simulink model "S1"  (R2023b)
settings: Solver=FixedStepAuto  StartTime=0.0  StopTime=Time-Step_T  FixedStep=Step_T  RelTol=1e-3
InitFcn:
  | run("P_sim.m")
values from neighbouring files (symbols this model uses):
  Step_T = 0.001    [P_sim.m]
  T = 0.1    [P_sim.m]
  x_1_0 = 0.2    [P_sim.m]
  x_2_0 = 0.5    [P_sim.m]
  x_3_0 = -1    [P_sim.m]
undefined symbols (not defined in the file or in its folder): pam
settings Model: Creator=admin  LastModifiedBy=admin

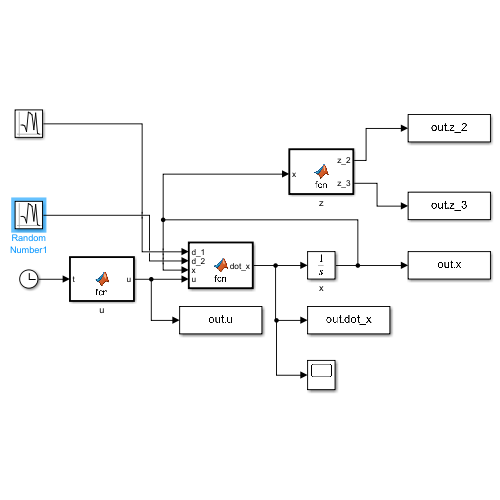
[thumbnail: Simulink's stored preview of the top-level diagram]
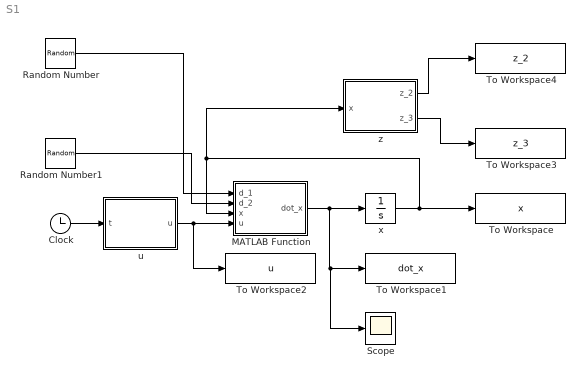
== system S1 ==
  Clock : Clock
  MATLAB Function : MATLAB Function  TreatAsAtomicUnit=on
  Random Number : RandomNumber  Variance=pam.d*pam.d  Seed=-1  SampleTime=Step_T
  Random Number1 : RandomNumber  Variance=pam.d*pam.d  Seed=1  SampleTime=Step_T
  Scope : Scope
  To Workspace : ToWorkspace  VariableName=x  SaveFormat=Timeseries  SampleTime=T
  To Workspace1 : ToWorkspace  VariableName=dot_x  SaveFormat=Timeseries  SampleTime=T
  To Workspace2 : ToWorkspace  VariableName=u  SaveFormat=Timeseries  SampleTime=T
  To Workspace3 : ToWorkspace  VariableName=z_3  SaveFormat=Timeseries  SampleTime=T
  To Workspace4 : ToWorkspace  VariableName=z_2  SaveFormat=Timeseries  SampleTime=T
  u : MATLAB Function  TreatAsAtomicUnit=on
  x : Integrator  InitialCondition=[x_1_0;x_2_0;x_3_0]
  z : MATLAB Function  TreatAsAtomicUnit=on
  wires:
  MATLAB Function/1(dot_x) -> Scope/1, To Workspace1/1, x/1
  x/1 -> To Workspace/1, MATLAB Function/3(x), z/1(x)
  u/1(u) -> To Workspace2/1, MATLAB Function/4(u)
  Clock/1 -> u/1(t)
  z/2(z_3) -> To Workspace3/1
  z/1(z_2) -> To Workspace4/1
  Random Number/1 -> MATLAB Function/1(d_1)
  Random Number1/1 -> MATLAB Function/2(d_2)

== matlab function S1/u ==
  data: t input; u output
function u  = fcn(t)

u = -0.5+t;

== matlab function S1/MATLAB Function ==
  data: d_1 input; d_2 input; x input; dot_x output; u input; pam parameter
function dot_x  = fcn(d_1,d_2,x,u,pam)

x_1 = x(1);
x_2 = x(2);
x_3 = x(3);

dot_x_1 = x_2;
dot_x_2 = x_3+pam.M/pam.D*sin(x_1)-pam.B/pam.D*x_2+d_1;
dot_x_3 = u+pam.K_m/pam.L*x_2-pam.J/pam.L*x_3+d_2;

dot_x = [dot_x_1;dot_x_2;dot_x_3];

== matlab function S1/z ==
  data: z_2 output; x input; z_3 output
function [z_2,z_3]  = fcn(x)

x_1 = x(1);
x_2 = x(2);
x_3 = x(3);

z_2 = [sin(x_1);x_2];
z_3 = [x_2;x_3];
